simulink model "tqdtqr_rebuild_V3"  (R2021b)
settings: Solver=VariableStepAuto  StartTime=0.0  StopTime=10.0  RelTol=1e-3
undefined symbols (not defined in the file): ATQD_AfterTqMinGain_X_Deg, ATQD_APSCreepBaseTqD_X_kph, ATQD_APSCreepBaseTqD_Y_Deg, ATQD_APSCreepBaseTqR_X_kph, ATQD_APSCreepBaseTqR_Y_Deg, ATQD_APSCreepIterm_X_kph, ATQD_APSCreepIterm_Y_kph, ATQD_APSCreepPterm_X_kph, ATQD_APSCreepPterm_Y_kph, ATQD_APSDecReq_X_kph, ATQD_APSDecReq_Y_mps2, ATQD_APSDecReqCMD_X_kph, ATQD_APSDecReqTs_X_pct, ATQD_APSDecTimeGain_X_Deg, ATQD_APSDecTimeGain_Y_s, ATQD_APSReqLowSpd_X_Deg, ATQD_AutoHoldReleaseBPS_X_Deg, ATQD_AWDLoadTrqnsGain_X_kg, ATQD_AWDLoadTrqnsGain_Y_pct, ATQD_BOSEnBPSPosn_X_kph, ATQD_BOSMap_X_rpm, ATQD_BOSMap_Y_pct, ATQD_CreepBaseTqD_X_kph, ATQD_CreepBaseTqD_Y_Deg, ATQD_CreepBaseTqR_X_kph, ATQD_CreepBaseTqR_Y_Deg, ATQD_CreepBPSDisPosn_X_Deg, ATQD_CreepBPSDisPosnR_X_Deg, ATQD_CreepBPSEnPosn_X_Deg, ATQD_CreepBPSEnPosnR_X_Deg, ATQD_CreepDeltaTq_X_kph, ATQD_CreepIterm_X_kph, ATQD_CreepIterm_Y_kph, ATQD_CreepItermMaxLimit_X_pct, ATQD_CreepPreloadTime_X_kph, ATQD_CreepPreloadTq_X_kph, ATQD_CreepPreloadTq_Y_s, ATQD_CreepProtTq_X_Deg, ATQD_CreepPterm_X_kph, ATQD_CreepPterm_Y_kph, ATQD_CreepRrTqSpRat_X_rpm, ATQD_CreepRrTqSpRat_Y_Nm, ATQD_CreepTargetSpdD_X_pct, ATQD_CreepTargetSpdR_X_pct, ATQD_CreepUpLimitTq_X_rpm, ATQD_DecIneOPDHoldEnDelay_X_Deg, ATQD_DecIneOPDHoldEnDelay_Y_bar, ATQD_ECOTqMapD_X_rpm, ATQD_ECOTqMapD_Y_pct, ATQD_EMTqMapD_X_rpm, ATQD_EMTqMapD_Y_pct, ATQD_EOPDTqMapDCon_X_rpm, ATQD_EOPDTqMapDCon_Y_Deg, ATQD_EstInitVehWeight_X_c, ATQD_FAfterTqCMDGain_X_rpm, ATQD_FAfterTqCMDGain_Y_pct, ATQD_ForceLowSpd_X_Deg, ATQD_ForcePLimitSpd_X_Deg, ATQD_FrLossMAPLowV_X_rpm, ATQD_FrLossMAPLowV_Y_Nm ... (+949)
libraries: simulink x235, hcu_lib x208, tqr x63, tqd x6
(part 17 of 37)

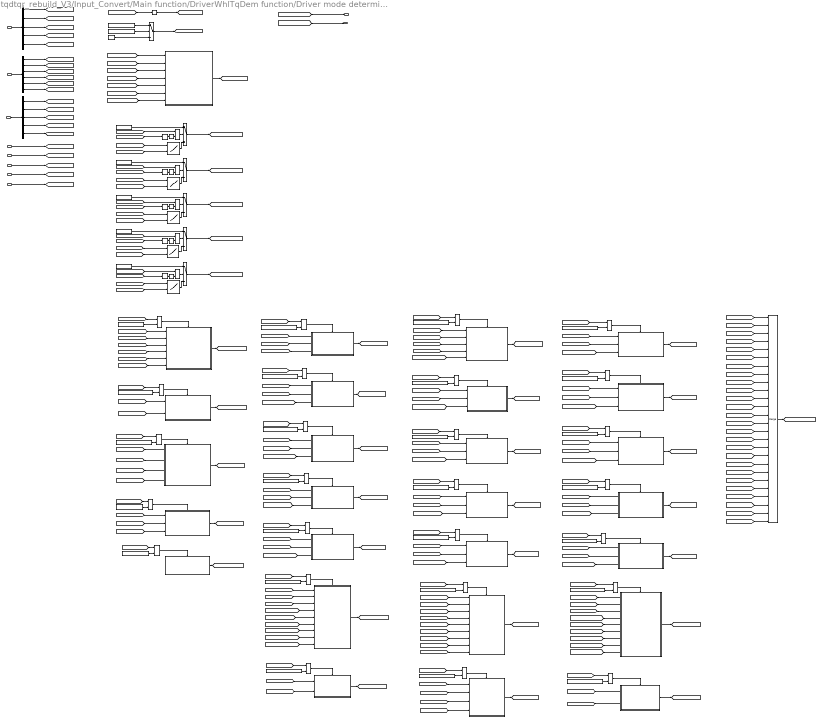
== system tqdtqr_rebuild_V3/Input_Convert/Main function/DriverWhlTqDem function/Driver mode determination ==
  note: No limp home shiftD sport LV1~5/OPD/invalid output Tq
  note: No limp home shiftD eco LV1~5/OPD/invalid output Tq
  note: No limp home shiftD normal LV1~5/OPD/invalid output Tq
  note: No limp home shiftR/N output Tq
  note: No limp home shiftD rock/snow output Tq
  note: Add road slope to output torque
  note: Output final torque
  note: Choose pedal map action(total 26 conditions)
  note: Limp home mode output Tq
  BSCPIn_outputs : Inport
  BSignalConvert_outputs : Inport  Port=2
  BFunction_outputs : Inport  Port=3
  VTQD_RollRegenEnable_flg : Inport  Port=4
  VTQD_RollingShaftSpd_rpm : Inport  Port=5
  VTQD_IVIRockModeEn_flg : Inport  Port=6
  VTQD_CreepEnable_flg : Inport  Port=7
  VTQD_PreDecTqLowLim_Nm : Inport  Port=8
  AND{8..12} (5 alike) : Logic  AllPortsSameDT=off  OutDataTypeStr=boolean
  Bus Selector : BusSelector  OutputSignals=VTQD_ActAPSPosn_pct,VTQD_LimpHomeAct_flg,VVMC_EstSlope_Deg,VINP_IVISnowModeCmd_flg,VDDM_VehMalfunLevel_enum
  Bus Selector1 : BusSelector  OutputSignals=VTQD_TqTargetShaftSpd_rpm,VTQD_EVDriveMode_enum,VTQD_RegenMode_enum,VTQD_LowIdleAccPedal_flg,VTQD_BrkSwSta_flg,VTQD_VehActSpd_kph
  Bus Selector2 : BusSelector  OutputSignals=VTQD_GearActualPosn_enum,VTQD_OPDHoldEnRel_flg,VTQD_APSReqTimer_s,VTQD_OPDHoldActRelTq_Nm,VTQD_DOALatchReq_flg
  Constant : Constant  Value=ENUM_PEDALMAPACTION_LHM
  Constant2 : Constant  Value=TRUE
  Constant3 : Constant  Value=KTQD_EVDriveModeValid_ovrdflg
  Constant35 : Constant  Value=ENUM_PEDALMAPACTION_NOLHMDROCK
  Constant36 : Constant  Value=ENUM_PEDALMAPACTION_NOLHMDSNOW
  Constant37 : Constant  Value=ENUM_PEDALMAPACTION_NOLHMN
  Constant38 : Constant  Value=ENUM_PEDALMAPACTION_NOLHMR
  Constant39 : Constant  Value=ENUM_PEDALMAPACTION_NOLHMDNRMLV1
  Constant40 : Constant  Value=ENUM_PEDALMAPACTION_NOLHMDNRMLV2
  Constant41 : Constant  Value=ENUM_PEDALMAPACTION_NOLHMDNRMLV3
  Constant42 : Constant  Value=ENUM_PEDALMAPACTION_NOLHMDNRMLV4
  Constant43 : Constant  Value=ENUM_PEDALMAPACTION_NOLHMDNRMLV5
  Constant44 : Constant  Value=ENUM_PEDALMAPACTION_NOLHMDNRMOPD
  Constant45 : Constant  Value=ENUM_PEDALMAPACTION_NOLHMDNRMINV
  Constant46 : Constant  Value=ENUM_PEDALMAPACTION_NOLHMDECOLV1
  Constant47 : Constant  Value=ENUM_PEDALMAPACTION_NOLHMDECOLV2
  Constant48 : Constant  Value=ENUM_PEDALMAPACTION_NOLHMDECOLV3
  Constant49 : Constant  Value=ENUM_PEDALMAPACTION_NOLHMDECOLV4
  Constant50 : Constant  Value=ENUM_PEDALMAPACTION_NOLHMDECOLV5
  Constant51 : Constant  Value=ENUM_PEDALMAPACTION_NOLHMDECOOPD
  Constant52 : Constant  Value=ENUM_PEDALMAPACTION_NOLHMDECOINV
  Constant53 : Constant  Value=ENUM_PEDALMAPACTION_NOLHMDSPORTLV1
  Constant54 : Constant  Value=ENUM_PEDALMAPACTION_NOLHMDSPORTLV2
  Constant55 : Constant  Value=ENUM_PEDALMAPACTION_NOLHMDSPORTLV3
  Constant56 : Constant  Value=ENUM_PEDALMAPACTION_NOLHMDSPORTLV4
  Constant57 : Constant  Value=ENUM_PEDALMAPACTION_NOLHMDSPORTLV5
  Constant58 : Constant  Value=ENUM_PEDALMAPACTION_NOLHMDSPORTOPD
  Constant59 : Constant  Value=ENUM_PEDALMAPACTION_NOLHMDSPORTINV
  Constant6 : Constant  Value=KTQD_EVDriveModeValid_ovrdval
  Constant{60..64} (5 alike) : Constant  Value=ZERO_FLOAT
  Delay{3..7} (5 alike) : Delay  DelayLength=1
  Equal{1..26} (26 alike) : RelationalOperator  Operator===  OutDataTypeStr=boolean  RndMeth=Simplest
  LHM : Subsystem
  MTQD_RL1TqMapDComp_Z_Nm : Lookup_n-D  BreakpointsForDimension1=ATQD_RL1TqMapDComp_Y_Deg  BreakpointsForDimension2=ATQD_RL1TqMapDComp_X_rpm  Table=MTQD_RL1TqMapDComp_Z_Nm  ExtrapMethod=Clip  InternalRulePriority=Speed  RndMeth=Simplest  InputSameDT=on
      settings: InputPortMap=u0,u1
  MTQD_RL2TqMapDComp_Z_Nm : Lookup_n-D  BreakpointsForDimension1=ATQD_RL1TqMapDComp_Y_Deg  BreakpointsForDimension2=ATQD_RL1TqMapDComp_X_rpm  Table=MTQD_RL2TqMapDComp_Z_Nm  ExtrapMethod=Clip  InternalRulePriority=Speed  RndMeth=Simplest  InputSameDT=on
      settings: InputPortMap=u0,u1
  MTQD_RL3TqMapDComp_Z_Nm : Lookup_n-D  BreakpointsForDimension1=ATQD_RL1TqMapDComp_Y_Deg  BreakpointsForDimension2=ATQD_RL1TqMapDComp_X_rpm  Table=MTQD_RL3TqMapDComp_Z_Nm  ExtrapMethod=Clip  InternalRulePriority=Speed  RndMeth=Simplest  InputSameDT=on
      settings: InputPortMap=u0,u1
  MTQD_RL4TqMapDComp_Z_Nm : Lookup_n-D  BreakpointsForDimension1=ATQD_RL1TqMapDComp_Y_Deg  BreakpointsForDimension2=ATQD_RL1TqMapDComp_X_rpm  Table=MTQD_RL4TqMapDComp_Z_Nm  ExtrapMethod=Clip  InternalRulePriority=Speed  RndMeth=Simplest  InputSameDT=on
      settings: InputPortMap=u0,u1
  MTQD_RL5TqMapDComp_Z_Nm : Lookup_n-D  BreakpointsForDimension1=ATQD_RL1TqMapDComp_Y_Deg  BreakpointsForDimension2=ATQD_RL1TqMapDComp_X_rpm  Table=MTQD_RL5TqMapDComp_Z_Nm  ExtrapMethod=Clip  InternalRulePriority=Speed  RndMeth=Simplest  InputSameDT=on
      settings: InputPortMap=u0,u1
  Merge : Merge  Inputs=26
  NOLHM ShiftD ECO Invalid : Subsystem
  "NOLHM ShiftD ECO LV1 " : Subsystem
  NOLHM ShiftD ECO LV2 : Subsystem
  NOLHM ShiftD ECO LV3 : Subsystem
  NOLHM ShiftD ECO LV4 : Subsystem
  NOLHM ShiftD ECO LV5 : Subsystem
  NOLHM ShiftD ECO OPD : Subsystem
  NOLHM ShiftD NRM Invalid : Subsystem
  NOLHM ShiftD NRM LV1 : Subsystem
  NOLHM ShiftD NRM LV2 : Subsystem
  NOLHM ShiftD NRM LV3 : Subsystem
  NOLHM ShiftD NRM LV4 : Subsystem
  NOLHM ShiftD NRM LV5 : Subsystem
  NOLHM ShiftD NRM OPD : Subsystem
  NOLHM ShiftD Sport Invalid : Subsystem
  NOLHM ShiftD Sport LV1 : Subsystem
  NOLHM ShiftD Sport LV2 : Subsystem
  NOLHM ShiftD Sport LV3 : Subsystem
  NOLHM ShiftD Sport LV4 : Subsystem
  NOLHM ShiftD Sport LV5 : Subsystem
  NOLHM ShiftD Sport OPD : Subsystem
  NOT{2..6} (5 alike) : Logic  Operator=NOT  AllPortsSameDT=off  OutDataTypeStr=boolean
  NoLHM ShiftD Rock : Subsystem
  NoLHM ShiftD Snow : Subsystem
  NoLHM ShiftProN : Subsystem
  NoLHM ShiftR : Subsystem
  Pedal map conditions decide : Stateflow chart  TreatAsAtomicUnit=on
  Relay1 : Relay  OnSwitchValue=KTQD_OPDHoldGradeUp_Deg  OffSwitchValue=KTQD_OPDHoldGradeDown_Deg  OnOutputValue=TRUE  OffOutputValue=FALSE  OutDataTypeStr=boolean
      settings: AttributesFormatString=|
      | ON:KTQD_OPDHoldGradeUp_Deg
      | OFF:KTQD_OPDHoldGradeDown_Deg
  Switch{,1..2,13..15} (6 alike) : Switch  Criteria=u2 ~= 0
      settings: AttributesFormatString=%<Criteria>
  VTQD_PedalMapWhlTqMerge_Nm : Outport
  VTQD_EVDriveModeValid_flg : Outport  Port=2
  wires:
  Constant2/1 -> Switch/3  "VTQD_EVDriveModeValid_flg"
  VTQD_RollingShaftSpd_rpm/1 -> [VTQD_RollingShaftSpd_rpm]
  [VVMC_EstSlope_Deg] -> Relay1/1
  Relay1/1 -> [VTQD_SlopeUp_flg]  "VTQD_SlopeUp_flg"
  Constant6/1 -> Switch/1
  Constant3/1 -> Switch/2
  Switch/1 -> [VTQD_EVDriveModeValid_flg]  "VTQD_EVDriveModeValid_flg"
  VTQD_CreepEnable_flg/1 -> [VTQD_CreepEnable_flg]
  [VTQD_LimpHomeAct_flg] -> Pedal map conditions decide/1(VTQD_LimpHomeAct_flg)
  [VTQD_EVDriveModeValid_flg] -> Pedal map conditions decide/2(VTQD_EVDriveModeValid_flg)
  [VTQD_GearActualPosn_enum] -> Pedal map conditions decide/3(VTQD_GearActualPosn_enum)
  [VTQD_IVIRockModeEn_flg] -> Pedal map conditions decide/4(VTQD_IVIRockModeEn_flg)
  [VINP_IVISnowModeCmd_flg] -> Pedal map conditions decide/5(VINP_IVISnowModeCmd_flg)
  [VTQD_EVDriveMode_enum] -> Pedal map conditions decide/6(VTQD_EVDriveMode_enum)
  [VTQD_RegenMode_enum] -> Pedal map conditions decide/7(VTQD_RegenMode_enum)
  Pedal map conditions decide/1(VTQD_PedalMapAction_enum) -> [VTQD_PedalMapAction_enum]
  [VTQD_PedalMapAction_enum] -> Equal1/1
  Constant/1 -> Equal1/2
  Equal1/1 -> LHM/Enable
  LHM/1(VTQD_PedalMapWhlTqLHM_Nm) -> [VTQD_PedalMapWhlTqLHM_Nm]
  [VTQD_PedalMapAction_enum] -> Equal2/1
  Equal2/1 -> NoLHM ShiftD Rock/Enable
  Constant35/1 -> Equal2/2
  NoLHM ShiftD Rock/1(VTQD_WhlTqRockMode_Nm) -> [VTQD_WhlTqRockMode_Nm]
  Constant36/1 -> Equal3/2
  [VTQD_PedalMapAction_enum] -> Equal3/1
  Equal3/1 -> NoLHM ShiftD Snow/Enable
  Equal4/1 -> NoLHM ShiftProN/Enable
  Constant37/1 -> Equal4/2
  [VTQD_PedalMapAction_enum] -> Equal4/1
  [VTQD_PedalMapAction_enum] -> Equal5/1
  Constant38/1 -> Equal5/2
  Equal5/1 -> NoLHM ShiftR/Enable
  Equal6/1 -> NOLHM ShiftD NRM LV1/Enable
  Constant39/1 -> Equal6/2
  [VTQD_PedalMapAction_enum] -> Equal6/1
  Constant40/1 -> Equal7/2
  [VTQD_PedalMapAction_enum] -> Equal7/1
  Equal7/1 -> NOLHM ShiftD NRM LV2/Enable
  [VTQD_PedalMapAction_enum] -> Equal8/1
  Equal8/1 -> NOLHM ShiftD NRM LV3/Enable
  Constant41/1 -> Equal8/2
  Equal9/1 -> NOLHM ShiftD NRM LV4/Enable
  [VTQD_PedalMapAction_enum] -> Equal9/1
  Constant42/1 -> Equal9/2
  Constant43/1 -> Equal10/2
  [VTQD_PedalMapAction_enum] -> Equal10/1
  Equal10/1 -> NOLHM ShiftD NRM LV5/Enable
  Equal11/1 -> NOLHM ShiftD NRM OPD/Enable
  [VTQD_PedalMapAction_enum] -> Equal11/1
  Constant44/1 -> Equal11/2
  Equal12/1 -> NOLHM ShiftD NRM Invalid/Enable
  [VTQD_PedalMapAction_enum] -> Equal12/1
  Constant45/1 -> Equal12/2
  Equal13/1 -> "NOLHM ShiftD ECO LV1 "/Enable
  Constant46/1 -> Equal13/2
  [VTQD_PedalMapAction_enum] -> Equal13/1
  [VTQD_PedalMapAction_enum] -> Equal14/1
  Constant47/1 -> Equal14/2
  Equal14/1 -> NOLHM ShiftD ECO LV2/Enable
  Constant48/1 -> Equal15/2
  Equal15/1 -> NOLHM ShiftD ECO LV3/Enable
  [VTQD_PedalMapAction_enum] -> Equal15/1
  [VTQD_PedalMapAction_enum] -> Equal16/1
  Equal16/1 -> NOLHM ShiftD ECO LV4/Enable
  Constant49/1 -> Equal16/2
  [VTQD_PedalMapAction_enum] -> Equal17/1
  Constant50/1 -> Equal17/2
  Equal17/1 -> NOLHM ShiftD ECO LV5/Enable
  Constant51/1 -> Equal18/2
  Equal18/1 -> NOLHM ShiftD ECO OPD/Enable
  [VTQD_PedalMapAction_enum] -> Equal18/1
  Equal19/1 -> NOLHM ShiftD ECO Invalid/Enable
  [VTQD_PedalMapAction_enum] -> Equal19/1
  Constant52/1 -> Equal19/2
  [VTQD_PedalMapAction_enum] -> Equal20/1
  Constant53/1 -> Equal20/2
  Equal20/1 -> NOLHM ShiftD Sport LV1/Enable
  Equal21/1 -> NOLHM ShiftD Sport LV2/Enable
  Constant54/1 -> Equal21/2
  [VTQD_PedalMapAction_enum] -> Equal21/1
  [VTQD_PedalMapAction_enum] -> Equal22/1
  Constant55/1 -> Equal22/2
  Equal22/1 -> NOLHM ShiftD Sport LV3/Enable
  Constant56/1 -> Equal23/2
  Equal23/1 -> NOLHM ShiftD Sport LV4/Enable
  [VTQD_PedalMapAction_enum] -> Equal23/1
  [VTQD_PedalMapAction_enum] -> Equal24/1
  Equal24/1 -> NOLHM ShiftD Sport LV5/Enable
  Constant57/1 -> Equal24/2
  [VTQD_PedalMapAction_enum] -> Equal25/1
  Equal25/1 -> NOLHM ShiftD Sport OPD/Enable
  Constant58/1 -> Equal25/2
  Constant59/1 -> Equal26/2
  Equal26/1 -> NOLHM ShiftD Sport Invalid/Enable
  [VTQD_PedalMapAction_enum] -> Equal26/1
  [VTQD_ActAPSPosn_pct] -> LHM/1(VTQD_ActAPSPosn_pct)
  [VTQD_TqTargetShaftSpd_rpm] -> LHM/2(VTQD_TqTargetShaftSpd_rpm)
  [VTQD_GearActualPosn_enum] -> LHM/3(VTQD_GearActualPosn_enum)
  [VDDM_VehMalfunLevel_enum] -> LHM/4(VDDM_VehMalfunLevel_enum)
  [VVMC_EstSlope_Deg] -> LHM/5(VVMC_EstSlope_Deg)
  [VTQD_VehActSpd_kph] -> LHM/6(VTQD_VehActSpd_kph)
  [VTQD_TqTargetShaftSpd_rpm] -> NoLHM ShiftD Rock/1(VTQD_TqTargetShaftSpd_rpm)
  [VTQD_ActAPSPosn_pct] -> NoLHM ShiftD Rock/2(VTQD_ActAPSPosn_pct)
  [VTQD_ActAPSPosn_pct] -> NoLHM ShiftD Snow/2(VTQD_ActAPSPosn_pct)
  [VTQD_PreDecTqLowLim_Nm] -> NoLHM ShiftD Snow/4(VTQD_PreDecTqLowLim_Nm)
  [VTQD_TqTargetShaftSpd_rpm] -> NoLHM ShiftD Snow/1(VTQD_TqTargetShaftSpd_rpm)
  [VTQD_RegenMode_enum] -> NoLHM ShiftD Snow/3(VTQD_RegenMode_enum)
  NoLHM ShiftD Snow/1(VTQD_WhlTqSnowMode_Nm) -> [VTQD_WhlTqSnowMode_Nm]
  [VTQD_TqTargetShaftSpd_rpm] -> NoLHM ShiftR/2(VTQD_TqTargetShaftSpd_rpm)
  [VTQD_ActAPSPosn_pct] -> NoLHM ShiftR/1(VTQD_ActAPSPosn_pct)
  NoLHM ShiftR/1(VTQD_PedalMapWhlTqR_Nm) -> [VTQD_PedalMapWhlTqR_Nm]
  NoLHM ShiftProN/1(VTQD_PedalMapWhlTqPorN_Nm) -> [VTQD_PedalMapWhlTqPorN_Nm]
  [VTQD_ActAPSPosn_pct] -> NOLHM ShiftD NRM LV1/1(VTQD_ActAPSPosn_pct)
  [VTQD_TqTargetShaftSpd_rpm] -> NOLHM ShiftD NRM LV1/2(VTQD_TqTargetShaftSpd_rpm)
  NOLHM ShiftD NRM LV1/1(VTQD_NL1TqMapDOut_Nm) -> [VTQD_NL1TqMapDOut_Nm]
  [VTQD_ActAPSPosn_pct] -> NOLHM ShiftD NRM LV2/1(VTQD_ActAPSPosn_pct)
  [VTQD_TqTargetShaftSpd_rpm] -> NOLHM ShiftD NRM LV2/2(VTQD_TqTargetShaftSpd_rpm)
  NOLHM ShiftD NRM LV2/1(VTQD_NL2TqMapDOut_Nm) -> [VTQD_NL2TqMapDOut_Nm]
  [VTQD_ActAPSPosn_pct] -> NOLHM ShiftD NRM LV3/1(VTQD_ActAPSPosn_pct)
  [VTQD_TqTargetShaftSpd_rpm] -> NOLHM ShiftD NRM LV3/2(VTQD_TqTargetShaftSpd_rpm)
  NOLHM ShiftD NRM LV3/1(VTQD_NL3TqMapDOut_Nm) -> [VTQD_NL3TqMapDOut_Nm]
  [VTQD_ActAPSPosn_pct] -> NOLHM ShiftD NRM LV4/1(VTQD_ActAPSPosn_pct)
  [VTQD_TqTargetShaftSpd_rpm] -> NOLHM ShiftD NRM LV4/2(VTQD_TqTargetShaftSpd_rpm)
  NOLHM ShiftD NRM LV4/1(VTQD_NL4TqMapDOut_Nm) -> [VTQD_NL4TqMapDOut_Nm]
  [VTQD_ActAPSPosn_pct] -> NOLHM ShiftD NRM LV5/1(VTQD_ActAPSPosn_pct)
  [VTQD_TqTargetShaftSpd_rpm] -> NOLHM ShiftD NRM LV5/2(VTQD_TqTargetShaftSpd_rpm)
  NOLHM ShiftD NRM LV5/1(VTQD_NL5TqMapDOut_Nm) -> [VTQD_NL5TqMapDOut_Nm]
  [VTQD_ActAPSPosn_pct] -> NOLHM ShiftD NRM OPD/1(VTQD_ActAPSPosn_pct)
  [VTQD_TqTargetShaftSpd_rpm] -> NOLHM ShiftD NRM OPD/2(VTQD_TqTargetShaftSpd_rpm)
  [VVMC_EstSlope_Deg] -> NOLHM ShiftD NRM OPD/3(VVMC_EstSlope_Deg)
  [VTQD_APSReqTimer_s] -> NOLHM ShiftD NRM OPD/4(VTQD_APSReqTimer_s)
  [VTQD_LowIdleAccPedal_flg] -> NOLHM ShiftD NRM OPD/5(VTQD_LowIdleAccPedal_flg)
  [VTQD_OPDHoldEnRel_flg] -> NOLHM ShiftD NRM OPD/6(VTQD_OPDHoldEnRel_flg)
  [VTQD_OPDHoldActRelTq_Nm] -> NOLHM ShiftD NRM OPD/7(VTQD_OPDHoldActRelTq_Nm)
  [VTQD_VehActSpd_kph] -> NOLHM ShiftD NRM OPD/8(VTQD_VehActSpd_kph)
  [VTQD_SlopeUp_flg] -> NOLHM ShiftD NRM OPD/9(VTQD_SlopeUp_flg)
  NOLHM ShiftD NRM OPD/1(VTQD_NOPDTqMapDOut_Nm) -> [VTQD_NOPDTqMapDOut_Nm]
  [VTQD_ActAPSPosn_pct] -> NOLHM ShiftD NRM Invalid/1(VTQD_ActAPSPosn_pct)
  [VTQD_TqTargetShaftSpd_rpm] -> NOLHM ShiftD NRM Invalid/2(VTQD_TqTargetShaftSpd_rpm)
  NOLHM ShiftD NRM Invalid/1(VTQD_NLTqMapDOutInv_Nm) -> [VTQD_NLTqMapDOutInv_Nm]
  [VTQD_RollRegenEnable_flg] -> "NOLHM ShiftD ECO LV1 "/1(VTQD_RollRegenEnable_flg)
  [VTQD_RollingShaftSpd_rpm] -> "NOLHM ShiftD ECO LV1 "/2(VTQD_RollingShaftSpd_rpm)
  [VTQD_TqTargetShaftSpd_rpm] -> "NOLHM ShiftD ECO LV1 "/3(VTQD_TqTargetShaftSpd_rpm)
  [VTQD_ActAPSPosn_pct] -> "NOLHM ShiftD ECO LV1 "/4(VTQD_ActAPSPosn_pct)
  "NOLHM ShiftD ECO LV1 "/1(VTQD_EL1TqMapDOut_Nm) -> [VTQD_EL1TqMapDOut_Nm]
  [VTQD_TqTargetShaftSpd_rpm] -> NOLHM ShiftD ECO LV2/2(VTQD_TqTargetShaftSpd_rpm)
  [VTQD_ActAPSPosn_pct] -> NOLHM ShiftD ECO LV2/1(VTQD_ActAPSPosn_pct)
  NOLHM ShiftD ECO LV2/1(VTQD_EL2TqMapDOut_Nm) -> [VTQD_EL2TqMapDOut_Nm]
  [VTQD_ActAPSPosn_pct] -> NOLHM ShiftD ECO LV3/1(VTQD_ActAPSPosn_pct)
  [VTQD_TqTargetShaftSpd_rpm] -> NOLHM ShiftD ECO LV3/2(VTQD_TqTargetShaftSpd_rpm)
  NOLHM ShiftD ECO LV3/1(VTQD_EL3TqMapDOut_Nm) -> [VTQD_EL3TqMapDOut_Nm]
  [VTQD_ActAPSPosn_pct] -> NOLHM ShiftD ECO LV4/1(VTQD_ActAPSPosn_pct)
  [VTQD_TqTargetShaftSpd_rpm] -> NOLHM ShiftD ECO LV4/2(VTQD_TqTargetShaftSpd_rpm)
  NOLHM ShiftD ECO LV4/1(VTQD_EL4TqMapDOut_Nm) -> [VTQD_EL4TqMapDOut_Nm]
  [VTQD_ActAPSPosn_pct] -> NOLHM ShiftD ECO LV5/1(VTQD_ActAPSPosn_pct)
  [VTQD_TqTargetShaftSpd_rpm] -> NOLHM ShiftD ECO LV5/2(VTQD_TqTargetShaftSpd_rpm)
  NOLHM ShiftD ECO LV5/1(VTQD_EL5TqMapDOut_Nm) -> [VTQD_EL5TqMapDOut_Nm]
  [VTQD_TqTargetShaftSpd_rpm] -> NOLHM ShiftD ECO OPD/2(VTQD_TqTargetShaftSpd_rpm)
  [VVMC_EstSlope_Deg] -> NOLHM ShiftD ECO OPD/3(VVMC_EstSlope_Deg)
  [VTQD_ActAPSPosn_pct] -> NOLHM ShiftD ECO OPD/1(VTQD_ActAPSPosn_pct)
  [VTQD_APSReqTimer_s] -> NOLHM ShiftD ECO OPD/4(VTQD_APSReqTimer_s)
  [VTQD_LowIdleAccPedal_flg] -> NOLHM ShiftD ECO OPD/5(VTQD_LowIdleAccPedal_flg)
  [VTQD_OPDHoldEnRel_flg] -> NOLHM ShiftD ECO OPD/6(VTQD_OPDHoldEnRel_flg)
  [VTQD_OPDHoldActRelTq_Nm] -> NOLHM ShiftD ECO OPD/7(VTQD_OPDHoldActRelTq_Nm)
  [VTQD_VehActSpd_kph] -> NOLHM ShiftD ECO OPD/8(VTQD_VehActSpd_kph)
  [VTQD_SlopeUp_flg] -> NOLHM ShiftD ECO OPD/9(VTQD_SlopeUp_flg)
  NOLHM ShiftD ECO OPD/1(VTQD_EOPDTqMapDOut_Nm) -> [VTQD_EOPDTqMapDOut_Nm]
  [VTQD_RollRegenEnable_flg] -> NOLHM ShiftD ECO Invalid/1(VTQD_RollRegenEnable_flg)
  [VTQD_RollingShaftSpd_rpm] -> NOLHM ShiftD ECO Invalid/2(VTQD_RollingShaftSpd_rpm)
  [VTQD_TqTargetShaftSpd_rpm] -> NOLHM ShiftD ECO Invalid/3(VTQD_TqTargetShaftSpd_rpm)
  [VTQD_ActAPSPosn_pct] -> NOLHM ShiftD ECO Invalid/4(VTQD_ActAPSPosn_pct)
  NOLHM ShiftD ECO Invalid/1(VTQD_ELTqMapDOutInv_Nm) -> [VTQD_ELTqMapDOutInv_Nm]
  [VTQD_ActAPSPosn_pct] -> NOLHM ShiftD Sport LV1/1(VTQD_ActAPSPosn_pct)
  [VTQD_TqTargetShaftSpd_rpm] -> NOLHM ShiftD Sport LV1/2(VTQD_TqTargetShaftSpd_rpm)
  NOLHM ShiftD Sport LV1/1(VTQD_SL1TqMapDOut_Nm) -> [VTQD_SL1TqMapDOut_Nm]
  [VTQD_ActAPSPosn_pct] -> NOLHM ShiftD Sport LV2/1(VTQD_ActAPSPosn_pct)
  [VTQD_TqTargetShaftSpd_rpm] -> NOLHM ShiftD Sport LV2/2(VTQD_TqTargetShaftSpd_rpm)
  NOLHM ShiftD Sport LV2/1(VTQD_SL2TqMapDOut_Nm) -> [VTQD_SL2TqMapDOut_Nm]
  [VTQD_ActAPSPosn_pct] -> NOLHM ShiftD Sport LV3/1(VTQD_ActAPSPosn_pct)
  [VTQD_TqTargetShaftSpd_rpm] -> NOLHM ShiftD Sport LV3/2(VTQD_TqTargetShaftSpd_rpm)
  NOLHM ShiftD Sport LV3/1(VTQD_SL3TqMapDOut_Nm) -> [VTQD_SL3TqMapDOut_Nm]
  [VTQD_ActAPSPosn_pct] -> NOLHM ShiftD Sport LV4/1(VTQD_ActAPSPosn_pct)
  [VTQD_TqTargetShaftSpd_rpm] -> NOLHM ShiftD Sport LV4/2(VTQD_TqTargetShaftSpd_rpm)
  NOLHM ShiftD Sport LV4/1(VTQD_SL4TqMapDOut_Nm) -> [VTQD_SL4TqMapDOut_Nm]
  [VTQD_ActAPSPosn_pct] -> NOLHM ShiftD Sport LV5/1(VTQD_ActAPSPosn_pct)
  [VTQD_TqTargetShaftSpd_rpm] -> NOLHM ShiftD Sport LV5/2(VTQD_TqTargetShaftSpd_rpm)
  NOLHM ShiftD Sport LV5/1(VTQD_SL5TqMapDOut_Nm) -> [VTQD_SL5TqMapDOut_Nm]
  [VTQD_ActAPSPosn_pct] -> NOLHM ShiftD Sport OPD/1(VTQD_ActAPSPosn_pct)
  [VTQD_TqTargetShaftSpd_rpm] -> NOLHM ShiftD Sport OPD/2(VTQD_TqTargetShaftSpd_rpm)
  [VVMC_EstSlope_Deg] -> NOLHM ShiftD Sport OPD/3(VVMC_EstSlope_Deg)
  [VTQD_APSReqTimer_s] -> NOLHM ShiftD Sport OPD/4(VTQD_APSReqTimer_s)
  [VTQD_LowIdleAccPedal_flg] -> NOLHM ShiftD Sport OPD/5(VTQD_LowIdleAccPedal_flg)
  [VTQD_OPDHoldEnRel_flg] -> NOLHM ShiftD Sport OPD/6(VTQD_OPDHoldEnRel_flg)
  [VTQD_OPDHoldActRelTq_Nm] -> NOLHM ShiftD Sport OPD/7(VTQD_OPDHoldActRelTq_Nm)
  [VTQD_VehActSpd_kph] -> NOLHM ShiftD Sport OPD/8(VTQD_VehActSpd_kph)
  [VTQD_SlopeUp_flg] -> NOLHM ShiftD Sport OPD/9(VTQD_SlopeUp_flg)
  NOLHM ShiftD Sport OPD/1(VTQD_SOPDTqMapDOut_Nm) -> [VTQD_SOPDTqMapDOut_Nm]
  [VTQD_ActAPSPosn_pct] -> NOLHM ShiftD Sport Invalid/1(VTQD_ActAPSPosn_pct)
  [VTQD_TqTargetShaftSpd_rpm] -> NOLHM ShiftD Sport Invalid/2(VTQD_TqTargetShaftSpd_rpm)
  NOLHM ShiftD Sport Invalid/1(VTQD_SLTqMapDOutInv_Nm) -> [VTQD_SLTqMapDOutInv_Nm]
  [VTQD_PedalMapWhlTqLHM_Nm] -> Merge/1
  [VTQD_WhlTqRockMode_Nm] -> Merge/2
  [VTQD_WhlTqSnowMode_Nm] -> Merge/3
  [VTQD_PedalMapWhlTqR_Nm] -> Merge/4
  [VTQD_PedalMapWhlTqPorN_Nm] -> Merge/5
  [VTQD_NL1TqMapDOut_Nm] -> Merge/6
  [VTQD_NL2TqMapDOut_Nm] -> Merge/7
  [VTQD_NL3TqMapDOut_Nm] -> Merge/8
  [VTQD_NL4TqMapDOut_Nm] -> Merge/9
  [VTQD_NL5TqMapDOut_Nm] -> Merge/10
  [VTQD_NOPDTqMapDOut_Nm] -> Merge/11
  [VTQD_NLTqMapDOutInv_Nm] -> Merge/12
  [VTQD_EL1TqMapDOut_Nm] -> Merge/13
  [VTQD_EL2TqMapDOut_Nm] -> Merge/14
  [VTQD_EL3TqMapDOut_Nm] -> Merge/15
  [VTQD_EL4TqMapDOut_Nm] -> Merge/16
  [VTQD_EL5TqMapDOut_Nm] -> Merge/17
  [VTQD_EOPDTqMapDOut_Nm] -> Merge/18
  [VTQD_ELTqMapDOutInv_Nm] -> Merge/19
  [VTQD_SL1TqMapDOut_Nm] -> Merge/20
  [VTQD_SL2TqMapDOut_Nm] -> Merge/21
  [VTQD_SL3TqMapDOut_Nm] -> Merge/22
  [VTQD_SL4TqMapDOut_Nm] -> Merge/23
  [VTQD_SL5TqMapDOut_Nm] -> Merge/24
  [VTQD_SOPDTqMapDOut_Nm] -> Merge/25
  [VTQD_SLTqMapDOutInv_Nm] -> Merge/26
  Merge/1 -> [VTQD_PedalMapWhlTqMerge_Nm]
  AND11/1 -> Switch14/2
  Constant62/1 -> Switch13/1
  AND10/1 -> Switch13/2
  [VTQD_CreepEnable_flg] -> Delay5/1
  [VTQD_TqTargetShaftSpd_rpm] -> MTQD_RL5TqMapDComp_Z_Nm/2
  NOT4/1 -> AND10/2
  [VTQD_BrkSwSta_flg] -> AND9/1
  NOT2/1 -> AND8/2
  AND8/1 -> Switch1/2
  [VTQD_TqTargetShaftSpd_rpm] -> MTQD_RL4TqMapDComp_Z_Nm/2
  [VVMC_EstSlope_Deg] -> MTQD_RL5TqMapDComp_Z_Nm/1
  NOT5/1 -> AND11/2
  [VTQD_TqTargetShaftSpd_rpm] -> MTQD_RL2TqMapDComp_Z_Nm/2
  [VVMC_EstSlope_Deg] -> MTQD_RL2TqMapDComp_Z_Nm/1
  [VTQD_TqTargetShaftSpd_rpm] -> MTQD_RL1TqMapDComp_Z_Nm/2
  [VVMC_EstSlope_Deg] -> MTQD_RL1TqMapDComp_Z_Nm/1
  Delay7/1 -> NOT2/1
  [VTQD_BrkSwSta_flg] -> AND10/1
  Delay3/1 -> NOT6/1
  [VTQD_CreepEnable_flg] -> Delay7/1
  Switch2/1 -> [VTQD_RL4TqMapDComp_Nm]  "VTQD_RL4TqMapDComp_Nm"
  NOT6/1 -> AND12/2
  Constant61/1 -> Switch2/1
  AND12/1 -> Switch15/2
  [VVMC_EstSlope_Deg] -> MTQD_RL3TqMapDComp_Z_Nm/1
  [VTQD_CreepEnable_flg] -> Delay3/1
  Constant60/1 -> Switch1/1
  Switch15/1 -> [VTQD_RL1TqMapDComp_Nm]  "VTQD_RL1TqMapDComp_Nm"
  Switch1/1 -> [VTQD_RL5TqMapDComp_Nm]  "VTQD_RL5TqMapDComp_Nm"
  AND9/1 -> Switch2/2
  MTQD_RL1TqMapDComp_Z_Nm/1 -> Switch15/3
  [VTQD_BrkSwSta_flg] -> AND12/1
  Switch14/1 -> [VTQD_RL2TqMapDComp_Nm]  "VTQD_RL2TqMapDComp_Nm"
  MTQD_RL5TqMapDComp_Z_Nm/1 -> Switch1/3
  [VVMC_EstSlope_Deg] -> MTQD_RL4TqMapDComp_Z_Nm/1
  MTQD_RL4TqMapDComp_Z_Nm/1 -> Switch2/3
  Constant63/1 -> Switch14/1
  MTQD_RL3TqMapDComp_Z_Nm/1 -> Switch13/3
  Delay4/1 -> NOT5/1
  [VTQD_BrkSwSta_flg] -> AND8/1
  [VTQD_CreepEnable_flg] -> Delay4/1
  Delay6/1 -> NOT3/1
  [VTQD_TqTargetShaftSpd_rpm] -> MTQD_RL3TqMapDComp_Z_Nm/2
  [VTQD_BrkSwSta_flg] -> AND11/1
  [VTQD_CreepEnable_flg] -> Delay6/1
  Delay5/1 -> NOT4/1
  MTQD_RL2TqMapDComp_Z_Nm/1 -> Switch14/3
  NOT3/1 -> AND9/2
  Constant64/1 -> Switch15/1
  Switch13/1 -> [VTQD_RL3TqMapDComp_Nm]  "VTQD_RL3TqMapDComp_Nm"
  [VTQD_RL1TqMapDComp_Nm] -> NOLHM ShiftD NRM LV1/3(VTQD_RL1TqMapDComp_Nm)
  [VTQD_RL2TqMapDComp_Nm] -> NOLHM ShiftD NRM LV2/3(VTQD_RL2TqMapDComp_Nm)
  [VTQD_RL3TqMapDComp_Nm] -> NOLHM ShiftD NRM LV3/3(VTQD_RL3TqMapDComp_Nm)
  [VTQD_RL4TqMapDComp_Nm] -> NOLHM ShiftD NRM LV4/3(VTQD_RL4TqMapDComp_Nm)
  [VTQD_RL5TqMapDComp_Nm] -> NOLHM ShiftD NRM LV5/3(VTQD_RL5TqMapDComp_Nm)
  [VTQD_RL1TqMapDComp_Nm] -> "NOLHM ShiftD ECO LV1 "/5(VTQD_RL1TqMapDComp_Nm)
  [VTQD_RL2TqMapDComp_Nm] -> NOLHM ShiftD ECO LV2/3(VTQD_RL2TqMapDComp_Nm)
  [VTQD_RL3TqMapDComp_Nm] -> NOLHM ShiftD ECO LV3/3(VTQD_RL3TqMapDComp_Nm)
  [VTQD_RL4TqMapDComp_Nm] -> NOLHM ShiftD ECO LV4/3(VTQD_RL4TqMapDComp_Nm)
  [VTQD_RL5TqMapDComp_Nm] -> NOLHM ShiftD ECO LV5/3(VTQD_RL5TqMapDComp_Nm)
  [VTQD_RL1TqMapDComp_Nm] -> NOLHM ShiftD Sport LV1/3(VTQD_RL1TqMapDComp_Nm)
  [VTQD_RL2TqMapDComp_Nm] -> NOLHM ShiftD Sport LV2/3(VTQD_RL2TqMapDComp_Nm)
  [VTQD_RL3TqMapDComp_Nm] -> NOLHM ShiftD Sport LV3/3(VTQD_RL3TqMapDComp_Nm)
  [VTQD_RL4TqMapDComp_Nm] -> NOLHM ShiftD Sport LV4/3(VTQD_RL4TqMapDComp_Nm)
  [VTQD_RL5TqMapDComp_Nm] -> NOLHM ShiftD Sport LV5/3(VTQD_RL5TqMapDComp_Nm)
  [VTQD_PedalMapWhlTqMerge_Nm] -> VTQD_PedalMapWhlTqMerge_Nm/1  "VTQD_PedalMapWhlTqMerge_Nm"
  BSCPIn_outputs/1 -> Bus Selector/1
  BSignalConvert_outputs/1 -> Bus Selector1/1
  BFunction_outputs/1 -> Bus Selector2/1
  Bus Selector2/1 -> [VTQD_GearActualPosn_enum]  "<VTQD_GearActualPosn_enum>"
  Bus Selector/1 -> [VTQD_ActAPSPosn_pct]  "<VTQD_ActAPSPosn_pct>"
  Bus Selector1/1 -> [VTQD_TqTargetShaftSpd_rpm]  "<VTQD_TqTargetShaftSpd_rpm>"
  Bus Selector/2 -> [VTQD_LimpHomeAct_flg]  "<VTQD_LimpHomeAct_flg>"
  Bus Selector1/2 -> [VTQD_EVDriveMode_enum]  "<VTQD_EVDriveMode_enum>"
  Bus Selector1/3 -> [VTQD_RegenMode_enum]  "<VTQD_RegenMode_enum>"
  VTQD_RollRegenEnable_flg/1 -> [VTQD_RollRegenEnable_flg]
  Bus Selector/3 -> [VVMC_EstSlope_Deg]  "<VVMC_EstSlope_Deg>"
  Bus Selector1/4 -> [VTQD_LowIdleAccPedal_flg]  "<VTQD_LowIdleAccPedal_flg>"
  Bus Selector1/5 -> [VTQD_BrkSwSta_flg]  "<VTQD_BrkSwSta_flg>"
  Bus Selector/4 -> [VINP_IVISnowModeCmd_flg]  "<VINP_IVISnowModeCmd_flg>"
  Bus Selector/5 -> [VDDM_VehMalfunLevel_enum]  "<VDDM_VehMalfunLevel_enum>"
  VTQD_PreDecTqLowLim_Nm/1 -> [VTQD_PreDecTqLowLim_Nm]
  [VTQD_EVDriveModeValid_flg] -> VTQD_EVDriveModeValid_flg/1
  Bus Selector1/6 -> [VTQD_VehActSpd_kph]  "<VTQD_VehActSpd_kph>"
  VTQD_IVIRockModeEn_flg/1 -> [VTQD_IVIRockModeEn_flg]
  Bus Selector2/4 -> [VTQD_OPDHoldActRelTq_Nm]  "<VTQD_OPDHoldActRelTq_Nm>"
  Bus Selector2/2 -> [VTQD_OPDHoldEnRel_flg]  "<VTQD_OPDHoldEnRel_flg>"
  Bus Selector2/3 -> [VTQD_APSReqTimer_s]  "<VTQD_APSReqTimer_s>"
  [VTQD_DOALatchReq_flg] -> NoLHM ShiftR/3(VTQD_DOALatchReq_flg)
  Bus Selector2/5 -> [VTQD_DOALatchReq_flg]  "<VTQD_DOALatchReq_flg>"

== system tqdtqr_rebuild_V3/Input_Convert/Main function/DriverWhlTqDem function/Low speed control ==
  BSCPIn_outputs : Inport
  BSignalConvert_outputs : Inport  Port=2
  AND15 : Logic  AllPortsSameDT=off  OutDataTypeStr=boolean
  AND16 : Logic  AllPortsSameDT=off  OutDataTypeStr=boolean
  AND6 : Logic  Inputs=4  AllPortsSameDT=off  OutDataTypeStr=boolean
  Bus Selector : BusSelector  OutputSignals=VVMC_LongAcc_Gps,VINP_VehSpeed_kph,VTQD_ActBPSPosn_pct,VINP_ADASAEBSta_enum,VTQD_LowIdleAccPedal_flg,task_time_s
  Bus Selector1 : BusSelector  OutputSignals=VTQD_BrkSwSta_flg,VTQD_VehActSpd_kph
  Constant : Constant  Value=KTQD_LoSpdCtrlBrkPos_pct
  Constant13 : Constant  Value=KTQD_EmergBrkSpd_kph
  Constant14 : Constant  Value=KTQD_EmergBrkLongAccel_Gps
  Constant15 : Constant  Value=ZERO_FLOAT
  Constant25 : Constant  Value=KTQD_LoSPdBrkRlsTime_s
  Constant26 : Constant  Value=KTQD_LoSpdBrkRlsSpd_kph
  Constant40 : Constant  Value=ENUM_ADASAEBSTA_ACTIVE
  Constant41 : Constant  Value=KTQD_AEBEmergBrkSpd_kph
  NOT : Logic  Operator=NOT  AllPortsSameDT=off  OutDataTypeStr=boolean
  NOT1 : Logic  Operator=NOT  AllPortsSameDT=off  OutDataTypeStr=boolean
  OR13 : Logic  Operator=OR  AllPortsSameDT=off  OutDataTypeStr=boolean
  OR2 : Logic  Operator=OR  AllPortsSameDT=off  OutDataTypeStr=boolean
  Relational Operator : RelationalOperator  OutDataTypeStr=boolean  RndMeth=Simplest
  Relational Operator{8..10,21} (4 alike) : RelationalOperator  Operator=<  OutDataTypeStr=boolean  RndMeth=Simplest
  Relational Operator20 : RelationalOperator  Operator===  OutDataTypeStr=boolean  RndMeth=Simplest
  Relational Operator6 : RelationalOperator  Operator=<=  OutDataTypeStr=boolean  RndMeth=Simplest
  Relational Operator7 : RelationalOperator  OutDataTypeStr=boolean  RndMeth=Simplest
  SR_Latch : hcu_lib/Basic_Blocks/SR_Latch
  Timer : hcu_lib/Basic_Blocks/Timer
  VTQD_LoSpdBrkCtrl_flg : Outport
  wires:
  Relational Operator7/1 -> OR2/2
  Relational Operator20/1 -> AND15/2
  Relational Operator10/1 -> AND16/1
  [VTQD_LowIdleAccPedal_flg] -> NOT/1
  [VVMC_LongAcc_Gps] -> Relational Operator8/1
  Constant13/1 -> Relational Operator10/2
  Constant40/1 -> Relational Operator20/2
  [VINP_VehSpeed_kph] -> Relational Operator21/1
  Constant41/1 -> Relational Operator21/2
  Constant15/1 -> Relational Operator9/2
  Relational Operator9/1 -> AND6/2
  Constant25/1 -> Relational Operator7/2, Timer/4
  Relational Operator21/1 -> AND15/1
  [task_time_s] -> Timer/3
  [VINP_ADASAEBSta_enum] -> Relational Operator20/1
  Relational Operator8/1 -> AND6/1
  OR2/1 -> SR_Latch/2  "VTQD_LoBrkCtrlReset_flg"
  AND16/1 -> OR13/1
  AND6/1 -> SR_Latch/1  "VTQD_TestLoSpdBrkCtrl_flg"
  [VTQD_ActBPSPosn_pct] -> Relational Operator/1
  Timer/1 -> Relational Operator7/1
  [VVMC_LongAcc_Gps] -> Relational Operator9/1
  NOT/1 -> OR2/1
  SR_Latch/1 -> [VTQD_LoSpdBrkCtrl_flg]  "VTQD_LoSpdBrkCtrl_flg"
  OR13/1 -> AND6/3
  Relational Operator6/1 -> Timer/1, NOT1/1
  Constant26/1 -> Relational Operator6/2
  AND15/1 -> OR13/2
  NOT1/1 -> Timer/2
  Constant14/1 -> Relational Operator8/2
  [VTQD_VehActSpd_kph] -> Relational Operator6/1
  Constant/1 -> Relational Operator/2
  [VTQD_BrkSwSta_flg] -> AND6/4
  [VINP_VehSpeed_kph] -> Relational Operator10/1
  Relational Operator/1 -> AND16/2
  BSCPIn_outputs/1 -> Bus Selector/1
  BSignalConvert_outputs/1 -> Bus Selector1/1
  Bus Selector/1 -> [VVMC_LongAcc_Gps]  "<VVMC_LongAcc_Gps>"
  Bus Selector/2 -> [VINP_VehSpeed_kph]  "<VINP_VehSpeed_kph>"
  Bus Selector/3 -> [VTQD_ActBPSPosn_pct]  "<VTQD_ActBPSPosn_pct>"
  Bus Selector/4 -> [VINP_ADASAEBSta_enum]  "<VINP_ADASAEBSta_enum>"
  Bus Selector1/1 -> [VTQD_BrkSwSta_flg]  "<VTQD_BrkSwSta_flg>"
  Bus Selector/5 -> [VTQD_LowIdleAccPedal_flg]  "<VTQD_LowIdleAccPedal_flg>"
  Bus Selector/6 -> [task_time_s]  "<task_time_s>"
  [VTQD_LoSpdBrkCtrl_flg] -> VTQD_LoSpdBrkCtrl_flg/1
  Bus Selector1/2 -> [VTQD_VehActSpd_kph]  "<VTQD_VehActSpd_kph>"

== system tqdtqr_rebuild_V3/Input_Convert/Main function/DriverWhlTqDem function/Pedal G-Control Mode ==
  BSCPIn_outputs : Inport
  BSignalConvert_outputs : Inport  Port=2
  BFunction_outputs : Inport  Port=3
  VTQD_CreepPrLoadEnable_flg : Inport  Port=4
  Active Determination : Subsystem
  Bus Selector : BusSelector  OutputSignals=VPMM_PowerSta_enum,VINP_SWC2RCustomizeSta_flg,task_time_s,VTQD_ActAPSPosn_pct,VVMC_LongAcc_Gps,VINP_VehSpeed_kph,VINP_BrkPedalPos_pct,VINP_SWCResUpSta_flg
  Bus Selector1 : BusSelector  OutputSignals=VTQD_RegenMode_enum,VTQD_TqTargetShaftSpd_rpm
  Bus Selector2 : BusSelector  OutputSignals=VTQD_SysMode_enum,VTQD_GearActualPosn_enum,VTQD_APSReqTimer_s
  Constant1 : Constant  Value=KTQD_IVICreepOnSW_flg
  Constant2 : Constant  Value=KTQD_IVIPedalGRegenLim_pct
  Constant3 : Constant  Value=KTQD_SmartRegenReq_mps2
  Constant4 : Constant  Value=KTQD_IVISmartRegenSW_flg
  Torque Calculation : Subsystem
  VTQD_PedAccTqEn_flg : Outport
  VTQD_PedalTqCal_Nm : Outport  Port=2
  wires:
  BSCPIn_outputs/1 -> Bus Selector/1
  BSignalConvert_outputs/1 -> Bus Selector1/1
  BFunction_outputs/1 -> Bus Selector2/1
  Bus Selector2/1 -> [VTQD_SysMode_enum]  "<VTQD_SysMode_enum>"
  Bus Selector/1 -> [VPMM_PwrSta_enum]  "<VPMM_PowerSta_enum>"
  Bus Selector2/2 -> [VTQD_GearActualPosn_enum]  "<VTQD_GearActualPosn_enum>"
  Bus Selector1/1 -> [VTQD_RegenMode_enum]  "<VTQD_RegenMode_enum>"
  Bus Selector/2 -> [VINP_SWC2RCustomizeSta_flg]  "<VINP_SWC2RCustomizeSta_flg>"
  Bus Selector/3 -> [task_time_s]  "<task_time_s>"
  Bus Selector/4 -> [VTQD_ActAPSPosn_pct]  "<VTQD_ActAPSPosn_pct>"
  Bus Selector1/2 -> [VTQD_TqTargetShaftSpd_rpm]  "<VTQD_TqTargetShaftSpd_rpm>"
  Bus Selector/5 -> [VVMC_LongAcc_Gps]  "<VVMC_LongAcc_Gps>"
  Bus Selector/6 -> [VINP_VehSpeed_kph]  "<VINP_VehSpeed_kph>"
  Bus Selector/7 -> [VINP_BrkPedalPos_pct]  "<VINP_BrkPedalPos_pct>"
  Bus Selector/8 -> [VINP_SWCResUpSta_flg]  "<VINP_SWCResUpSta_flg>"
  [VTQD_PedAccTqEn_flg] -> VTQD_PedAccTqEn_flg/1
  [VTQD_PedalTqCal_Nm] -> VTQD_PedalTqCal_Nm/1
  [VTQD_APSReqTimer_s] -> Torque Calculation/13(VTQD_APSReqTimer_s)
  [VINP_SWCResUpSta_flg] -> Active Determination/7(VINP_SWCResUpSta_flg)
  Constant3/1 -> Torque Calculation/10(VVMC_SmartRegenReq_mps2)  "VTQD_SmartRegenReq_mps2"
  Constant1/1 -> Torque Calculation/12(VINP_IVICreepOnSW_flg)  "VTQD_IVICreepOnSW_flg"
  [VTQD_ActAPSPosn_pct] -> Torque Calculation/1(VTQD_ActAPSPosn_pct)
  [VPMM_PwrSta_enum] -> Active Determination/2(VPMM_PwrSta_enum)
  [VTQD_TqTargetShaftSpd_rpm] -> Torque Calculation/2(VTQD_TqTargetShaftSpd_rpm)
  [task_time_s] -> Active Determination/6(task_time_s)
  [VTQD_GearActualPosn_enum] -> Torque Calculation/6(VTQD_GearActualPosn_enum)
  [VTQD_CreepPrLoadEnable_flg] -> Torque Calculation/7(VTQD_CreepPrLoadEnable_flg)
  [VINP_BrkPedalPos_pct] -> Torque Calculation/8(VINP_BrkPedalPos_pct)
  [VINP_SWC2RCustomizeSta_flg] -> Active Determination/5(VINP_SWC2RCustomizeSta_flg)
  [VINP_VehSpeed_kph] -> Torque Calculation/4(VINP_VehSpeed_kph)
  Constant4/1 -> Torque Calculation/11(VINP_IVISmartRegenSW_flg)  "VTQD_IVISmartRegenSW_flg"
  [VTQD_SysMode_enum] -> Active Determination/1(VINP_SCPSystemMode_enum)
  [VTQD_PedAccTqEn_flg] -> Torque Calculation/5(VTQD_PedAccTqEn_flg)
  [VVMC_LongAcc_Gps] -> Torque Calculation/3(VVMC_LongAcc_Gps)
  [VTQD_RegenMode_enum] -> Active Determination/4(VTQD_RegenMode_enum)
  [VTQD_GearActualPosn_enum] -> Active Determination/3(VTQD_GearActualPosn_enum)
  Torque Calculation/1(VTQD_PedalTqCal_Nm) -> [VTQD_PedalTqCal_Nm]
  Active Determination/1(VTQD_PedAccTqEn_flg) -> [VTQD_PedAccTqEn_flg]
  Constant2/1 -> Torque Calculation/9(VINP_IVIPedalGRegenLim_pct)  "VTQD_IVIPedalGRegenLim_pct"
  VTQD_CreepPrLoadEnable_flg/1 -> [VTQD_CreepPrLoadEnable_flg]
  Bus Selector2/3 -> [VTQD_APSReqTimer_s]  "<VTQD_APSReqTimer_s>"
